simulink model "task1simulink"  (R2016a)
settings: Solver=FixedStepAuto  StartTime=0.0  StopTime=inf  FixedStep=1  RelTol=1e-3
undefined symbols (not defined in the file): Header
libraries: robotlib x3
settings Model: Creator=sprinkle  LastModifiedBy=sprinkle
settings OptimizationCC: OptimizeModelRefInitCode=on  LifeSpan=Inf  MaxStackSize=64
settings HardwareCC: ProdBitPerPointer=32  ProdLargestAtomicFloat=None  ProdIntDivRoundTo=Undefined  ProdEndianess=Unspecified  ProdWordSize=32  ProdHWDeviceType=Generic->Unspecified (assume 32-bit Generic)
settings RTWCC: SystemTargetFile=ert.tlc  HardwareBoard=Robot Operating System (ROS)  TemplateMakefile=ert_default_tmf  GenerateReport=on  Toolchain=Catkin  IncludeHyperlinkInReport=on  LaunchReport=on  TargetLang=C++  GenerateTraceInfo=on  GenerateTraceReport=on  GenerateTraceReportSl=on  GenerateTraceReportSf=on  GenerateTraceReportEml=on
settings CodeAppCC: ForceParamTrailComments=on  IgnoreCustomStorageClasses=off  OperatorAnnotations=on  SimulinkDataObjDesc=on  SFDataObjDesc=on  MATLABFcnDesc=on  InsertBlockDesc=on  MATLABSourceComments=on

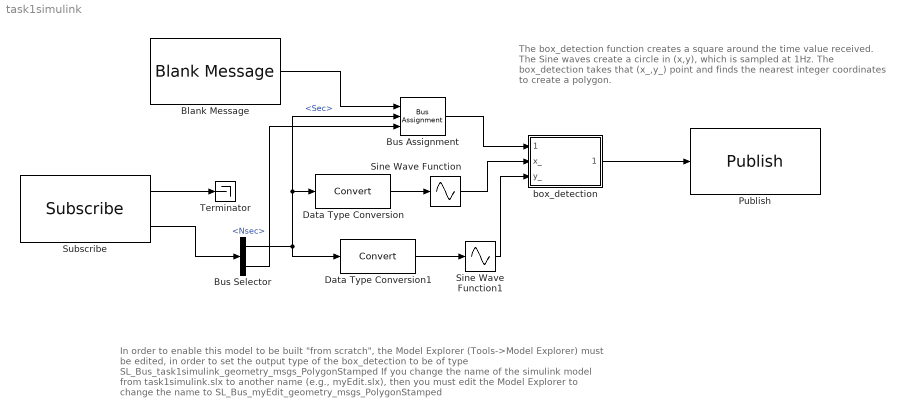
== system task1simulink ==
  note: In order to enable this model to be built "from scratch", the Model Explorer (Tools->Model Explorer) must be
      | edited, in order to set the output type of the box_detection to be of type
      | SL_Bus_task1simulink_geometry_msgs_PolygonStamped
      | If you change the name of the simulink model from task1simulink.slx to another name (e.g., myEdit.slx),
      | then you must edit the Model Explorer to change the name to
      | SL_Bus_myEdit_geometry_msgs_PolygonStamped
  note: The box_detection function creates a square around the time
      | value received. The Sine waves create a circle in (x,y), which
      | is sampled at 1Hz. The box_detection takes that (x_,y_) point
      | and finds the nearest integer coordinates to create a polygon.
  Blank Message : robotlib/Blank Message  SourceLibraryInfo=This block requires Robotics System Toolbox  messageType=geometry_msgs/PolygonStamped  SampleTime=inf
  Bus Assignment : BusAssignment  AssignedSignals=Header.Stamp.Sec,Header.Stamp.Nsec
  Bus Selector : BusSelector  OutputSignals=Clock_.Sec,Clock_.Nsec
  Data Type Conversion : DataTypeConversion
  Data Type Conversion1 : DataTypeConversion
  Publish : robotlib/Publish  SourceLibraryInfo=This block requires Robotics System Toolbox  topicSource=Specify your own  topic=/detections  messageType=geometry_msgs/PolygonStamped  messageQueueLength=1
  Sine Wave Function : Sin  TimeSource=Use external signal  Amplitude=3  Frequency=0.2  SampleTime=0
  Sine Wave Function1 : Sin  TimeSource=Use external signal  Amplitude=3  Frequency=0.2  Phase=pi/2  SampleTime=0
  Subscribe : robotlib/Subscribe  SourceLibraryInfo=This block requires Robotics System Toolbox  topicSource=Select from ROS network  topic=/clock  messageType=rosgraph_msgs/Clock  sampleTime=-1  messageQueueLength=1
  Terminator : Terminator
  box_detection : MATLAB Function  TreatAsAtomicUnit=on
  wires:
  Blank Message/1 -> Bus Assignment/1
  box_detection/1(outputMsg) -> Publish/1
  Bus Assignment/1 -> box_detection/1(blankMsg)
  Sine Wave Function/1 -> box_detection/2(x_)
  Sine Wave Function1/1 -> box_detection/3(y_)
  Subscribe/1 -> Terminator/1
  Subscribe/2 -> Bus Selector/1
  Bus Selector/1 -> Data Type Conversion/1, Bus Assignment/2, Data Type Conversion1/1  "<Sec>"
  Bus Selector/2 -> Bus Assignment/3  "<Nsec>"
  Data Type Conversion/1 -> Sine Wave Function/1
  Data Type Conversion1/1 -> Sine Wave Function1/1

== matlab function task1simulink/box_detection ==
  data: blankMsg input; x_ input; outputMsg output Bus: SL_Bus_task1simulink_geometry_msgs_PolygonStamped; y_ input
    function outputMsg = fcn(blankMsg,x_,y_)
    %#codegen
    % the sequence of the message must increment each time we publish, so we
    % need it to be persistent across instantiations
    persistent seq;

    % if this is the first time our model is run, then 'seq' will not exist.
    % Then 'isempty(seq)' will be true, which allows us to intialize it to 0
    if isempty(seq)
        seq=uint32(0);
    end

    % increment the sequence number
    seq = seq+1;
    % set our output to be a copy of the input (blankMsg)
    outputMsg = blankMsg;
    % these points in (x,y,z) are either taken from the inputs, or hardcoded
    x = single(x_);
    y = single(y_);
    z = single(0);
    % by definition in this block, we are making a square.
    % IF YOU USE THIS model as inspiration for an output detection that is a
    % pentagon, then you would set the length to be 5, for example.
    outputMsg.Polygon.Points_SL_Info.CurrentLength = uint32(4);
    % set the frame to be relative to our base of 0. If you want to use data
    % coming from another detection, then you can set the /detections to be in
    % the frame of that specific sensor
    str = 'catvehicle/odom';
    % initialize the header and set its values
    strLength = length(str);
    outputMsg.Header.Seq = seq;
    outputMsg.Header.FrameId(1:strLength) = str;
    outputMsg.Header.FrameId_SL_Info.CurrentLength = uint32(strLength);

    % populate point 1
    outputMsg.Polygon.Points(1).X = floor(x);
    outputMsg.Polygon.Points(1).Y = floor(y);
    outputMsg.Polygon.Points(1).Z = z;

    % populate point 2
    outputMsg.Polygon.Points(2).X = floor(x);
    outputMsg.Polygon.Points(2).Y = ceil(y);
    outputMsg.Polygon.Points(2).Z = z;

    % populate point 3
    outputMsg.Polygon.Points(3).X = ceil(x);
    outputMsg.Polygon.Points(3).Y = ceil(y);
    outputMsg.Polygon.Points(3).Z = z;

    % populate point 4
    outputMsg.Polygon.Points(4).X = ceil(x);
    outputMsg.Polygon.Points(4).Y = floor(y);
    outputMsg.Polygon.Points(4).Z = z;

    % note that the polygon type "closes" between the last and first points
